simulink model "Assignment2_NaturalPulseDetect"  (R2017b)
settings: Solver=FixedStepAuto  StartTime=0.0  StopTime=inf  FixedStep=0.001  RelTol=1e-3  EnableMultiTasking=on
undefined symbols (not defined in the file): D0, D1, D10, D11, D12, D13, D2, D3, D5, D6, D8, D9, PTA0, PTA1, PTA2, PTB9, PTC16, PTC17, PTC2, PTC4, PTD0, PTD1, PTD2, PTD3
libraries: frdmk64flib x28, etargetslib x7
settings Model: ExtModeTrigDuration=5  Creator=montema2  LastModifiedBy=farona
settings OptimizationCC: PassReuseOutputArgsAs=Individual arguments  MaxStackSize=64
settings DebuggingCC: ParameterTunabilityLossMsg=error
settings HardwareCC: ProdBitPerPointer=32  ProdBitPerSizeT=32  ProdBitPerPtrDiffT=32  ProdLargestAtomicInteger=Long  ProdLargestAtomicFloat=Double  ProdWordSize=32  ProdHWDeviceType=ARM Compatible->ARM Cortex
settings SFSimCC: MATLABDynamicMemAlloc=off
settings RTWCC: SystemTargetFile=ert.tlc  HardwareBoard=NXP FRDM-K64F  TemplateMakefile=ert_default_tmf  GenerateReport=on  Toolchain=GNU Tools for ARM Embedded Processors  IncludeHyperlinkInReport=on  LaunchReport=on  GenerateTraceInfo=on  GenerateTraceReport=on  GenerateTraceReportSl=on  GenerateTraceReportSf=on  GenerateTraceReportEml=on
settings CodeAppCC: ForceParamTrailComments=on  IgnoreCustomStorageClasses=off  OperatorAnnotations=on  SimulinkDataObjDesc=on  SFDataObjDesc=on  InsertBlockDesc=on

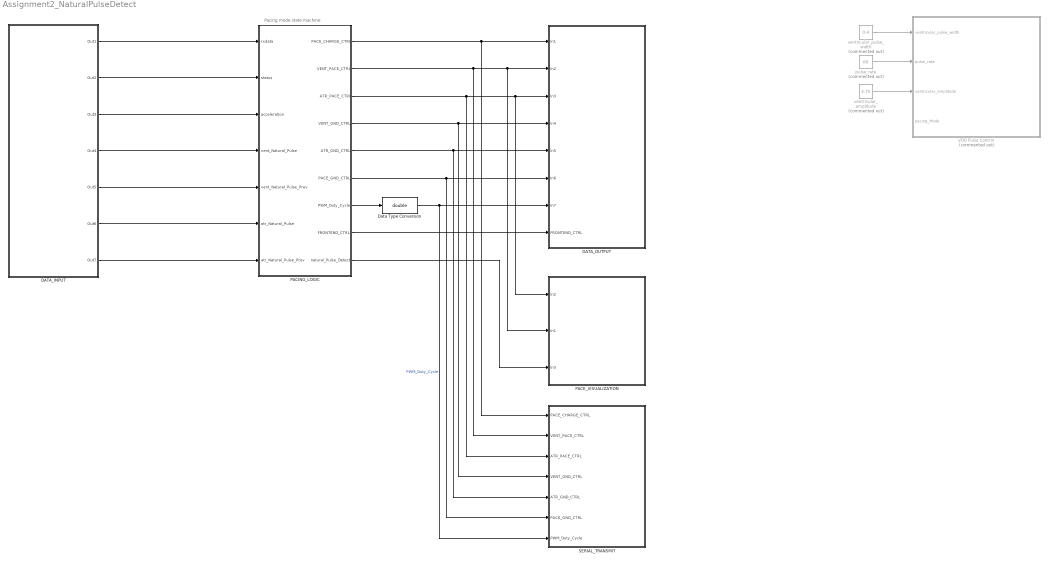
== system Assignment2_NaturalPulseDetect ==
  note: Pacing mode state machine
  DATA_INPUT : Subsystem
  DATA_OUTPUT : Subsystem
  Data Type Conversion : DataTypeConversion  OutDataTypeStr=double  RndMeth=Nearest
  PACE_VISUALIZATION : Subsystem
  PACING_LOGIC : Stateflow chart  TreatAsAtomicUnit=on
  SERIAL_TRANSMIT : Subsystem
  VOO Pulse Control : Subsystem  Commented=on
  pulse_rate : Constant  Commented=on  Value=60  OutMin=[50]  OutMax=[175]
  ventricular_amplitude : Constant  Commented=on  Value=3.75
  ventricular_pulse_width : Constant  Commented=on  Value=0.4
  wires:
  ventricular_pulse_width/1 -> VOO Pulse Control/1(ventricular_pulse_width)
  pulse_rate/1 -> VOO Pulse Control/2(pulse_rate)
  ventricular_amplitude/1 -> VOO Pulse Control/3(ventricular_amplitude)
  PACING_LOGIC/4(VENT_GND_CTRL) -> SERIAL_TRANSMIT/4(VENT_GND_CTRL), DATA_OUTPUT/4(In4)
  PACING_LOGIC/6(PACE_GND_CTRL) -> SERIAL_TRANSMIT/6(PACE_GND_CTRL), DATA_OUTPUT/6(In6)
  PACING_LOGIC/1(PACE_CHARGE_CTRL) -> SERIAL_TRANSMIT/1(PACE_CHARGE_CTRL), DATA_OUTPUT/1(In1)
  PACING_LOGIC/7(PWM_Duty_Cycle) -> Data Type Conversion/1
  PACING_LOGIC/5(ATR_GND_CTRL) -> SERIAL_TRANSMIT/5(ATR_GND_CTRL), DATA_OUTPUT/5(In5)
  PACING_LOGIC/2(VENT_PACE_CTRL) -> SERIAL_TRANSMIT/2(VENT_PACE_CTRL), PACE_VISUALIZATION/2(In1), DATA_OUTPUT/2(In2)
  PACING_LOGIC/3(ATR_PACE_CTRL) -> SERIAL_TRANSMIT/3(ATR_PACE_CTRL), PACE_VISUALIZATION/1(In2), DATA_OUTPUT/3(In3)
  PACING_LOGIC/9(natural_Pulse_Detect) -> PACE_VISUALIZATION/3(In3)
  Data Type Conversion/1 -> SERIAL_TRANSMIT/7(PWM_Duty_Cycle), DATA_OUTPUT/7(In7)  "PWM_Duty_Cycle"
  PACING_LOGIC/8(FRONTEND_CTRL) -> DATA_OUTPUT/8(FRONTEND_CTRL)
  DATA_INPUT/1(Out1) -> PACING_LOGIC/1(rxdata)
  DATA_INPUT/2(Out2) -> PACING_LOGIC/2(status)
  DATA_INPUT/3(Out3) -> PACING_LOGIC/3(acceleration)
  DATA_INPUT/4(Out4) -> PACING_LOGIC/4(vent_Natural_Pulse)
  DATA_INPUT/5(Out5) -> PACING_LOGIC/5(vent_Natural_Pulse_Prev)
  DATA_INPUT/6(Out6) -> PACING_LOGIC/6(atr_Natural_Pulse)
  DATA_INPUT/7(Out7) -> PACING_LOGIC/7(atr_Natural_Pulse_Prev)

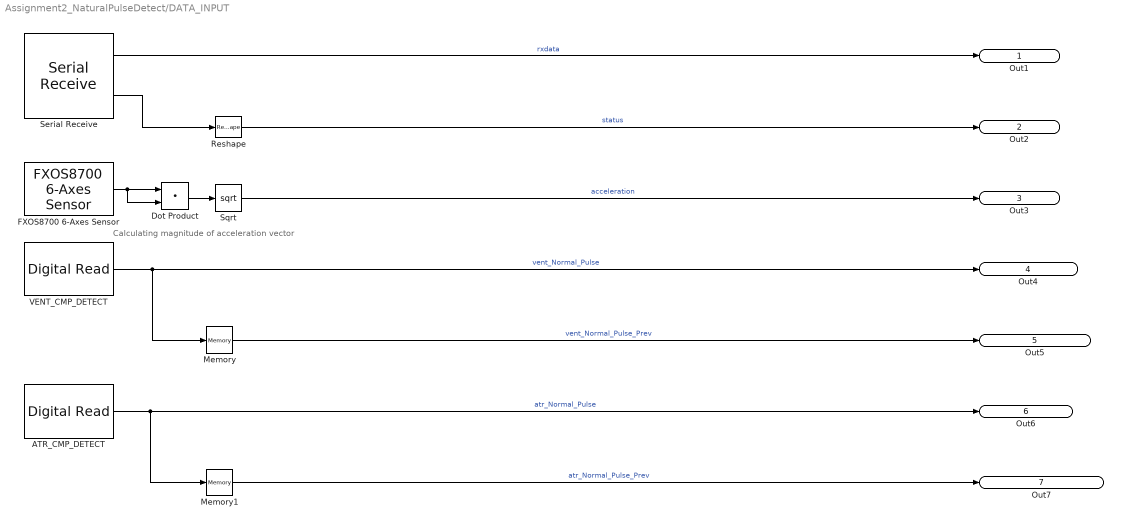
== system Assignment2_NaturalPulseDetect/DATA_INPUT ==
  note: Calculating magnitude of acceleration vector
  ATR_CMP_DETECT : frdmk64flib/Digital Read  Whichpin=PTC16 (D0)  SampleTime=-1
      settings: SourceProductName=Simulink Coder Support Package for NXP FRDM-K64F Board
  Dot Product : DotProduct  InputSameDT=on  OutDataTypeStr=Inherit: Inherit via internal rule
  FXOS8700 6-Axes Sensor : frdmk64flib/FXOS8700 6-Axes Sensor  Activesensor=Accelerometer only  ODR=800Hz  HybridODR=400Hz  Accelfullrange=-2g to +2g  SampleTime=-1
      settings: SourceProductName=Simulink Coder Support Package for NXP FRDM-K64F Board
  Memory : Memory
  Memory1 : Memory
  Reshape : Reshape  OutputDimensionality=Customize  OutputDimensions=[1]
  Serial Receive : frdmk64flib/Serial Receive  SCIModule=0  Baudrate=uint32(9600)  Parity=None  StopBits=1  HardwareFlowControl=None  ByteOrder=LittleEndian  DataType=uint8  DataLength=44  BlockingMode=off  OutputStatus=on  SampleTime=-1
      settings: SourceProductName=Simulink Coder Support Package for NXP FRDM-K64F Board
  Sqrt : Sqrt  SaturateOnIntegerOverflow=on
  VENT_CMP_DETECT : frdmk64flib/Digital Read  Whichpin=PTC17 (D1)  SampleTime=-1
      settings: SourceProductName=Simulink Coder Support Package for NXP FRDM-K64F Board
  Out1 : Outport
  Out2 : Outport  Port=2
  Out3 : Outport  Port=3
  Out4 : Outport  Port=4
  Out5 : Outport  Port=5
  Out6 : Outport  Port=6
  Out7 : Outport  Port=7
  wires:
  Serial Receive/2 -> Reshape/1
  Serial Receive/1 -> Out1/1  "rxdata"
  Dot Product/1 -> Sqrt/1
  FXOS8700 6-Axes Sensor/1 -> Dot Product/2, Dot Product/1
  Reshape/1 -> Out2/1  "status"
  Sqrt/1 -> Out3/1  "acceleration"
  VENT_CMP_DETECT/1 -> Out4/1, Memory/1  "vent_Normal_Pulse"
  Memory/1 -> Out5/1  "vent_Normal_Pulse_Prev"
  Memory1/1 -> Out7/1  "atr_Normal_Pulse_Prev"
  ATR_CMP_DETECT/1 -> Out6/1, Memory1/1  "atr_Normal_Pulse"

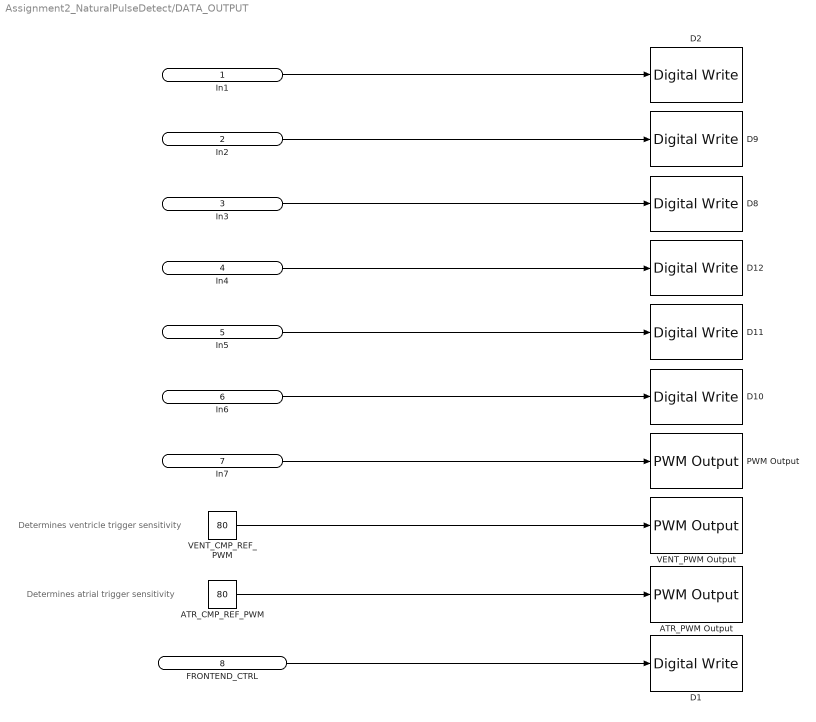
== system Assignment2_NaturalPulseDetect/DATA_OUTPUT ==
  note: Determines ventricle trigger sensitivity
  note: Determines atrial trigger sensitivity
  In1 : Inport
  In2 : Inport  Port=2
  In3 : Inport  Port=3
  In4 : Inport  Port=4
  In5 : Inport  Port=5
  In6 : Inport  Port=6
  In7 : Inport  Port=7
  FRONTEND_CTRL : Inport  Port=8
  ATR_CMP_REF_PWM : Constant  Value=80
  ATR_PWM Output : frdmk64flib/PWM Output  Whichpin=PTC2 (D6)  InitialFrequency=1000  InitialDutyCycle=0
      settings: SourceProductName=Simulink Coder Support Package for NXP FRDM-K64F Board
  D1 : frdmk64flib/Digital Write  Whichpin=PTD1 (D13)
      settings: SourceProductName=Simulink Coder Support Package for NXP FRDM-K64F Board
  D10 : frdmk64flib/Digital Write  Whichpin=PTD0 (D10)
      settings: SourceProductName=Simulink Coder Support Package for NXP FRDM-K64F Board
  D11 : frdmk64flib/Digital Write  Whichpin=PTD2 (D11)
      settings: SourceProductName=Simulink Coder Support Package for NXP FRDM-K64F Board
  D12 : frdmk64flib/Digital Write  Whichpin=PTD3 (D12)
      settings: SourceProductName=Simulink Coder Support Package for NXP FRDM-K64F Board
  D2 : frdmk64flib/Digital Write  Whichpin=PTB9 (D2)
      settings: SourceProductName=Simulink Coder Support Package for NXP FRDM-K64F Board
  D8 : frdmk64flib/Digital Write  Whichpin=PTA0 (D8)
      settings: SourceProductName=Simulink Coder Support Package for NXP FRDM-K64F Board
  D9 : frdmk64flib/Digital Write  Whichpin=PTC4 (D9)
      settings: SourceProductName=Simulink Coder Support Package for NXP FRDM-K64F Board
  PWM Output : frdmk64flib/PWM Output  Whichpin=PTA2 (D5)  InitialFrequency=1000  InitialDutyCycle=0
      settings: SourceProductName=Simulink Coder Support Package for NXP FRDM-K64F Board
  VENT_CMP_REF_PWM : Constant  Value=80
  VENT_PWM Output : frdmk64flib/PWM Output  Whichpin=PTA1 (D3)  InitialFrequency=1000  InitialDutyCycle=0
      settings: SourceProductName=Simulink Coder Support Package for NXP FRDM-K64F Board
  wires:
  In1/1 -> D2/1
  In6/1 -> D10/1
  In2/1 -> D9/1
  In4/1 -> D12/1
  In3/1 -> D8/1
  In7/1 -> PWM Output/1
  In5/1 -> D11/1
  VENT_CMP_REF_PWM/1 -> VENT_PWM Output/1
  FRONTEND_CTRL/1 -> D1/1
  ATR_CMP_REF_PWM/1 -> ATR_PWM Output/1

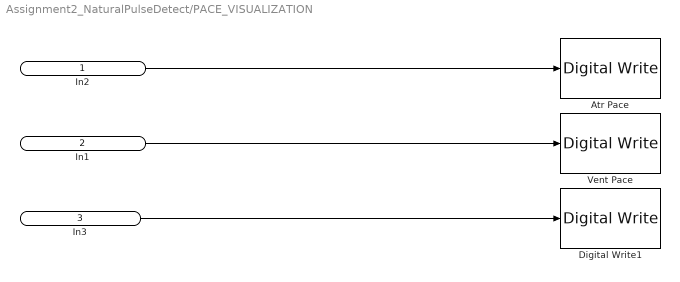
== system Assignment2_NaturalPulseDetect/PACE_VISUALIZATION ==
  In2 : Inport
  In1 : Inport  Port=2
  In3 : Inport  Port=3
  Atr Pace : frdmk64flib/Digital Write  Whichpin=GREEN_LED
      settings: SourceProductName=Simulink Coder Support Package for NXP FRDM-K64F Board
  Digital Write1 : frdmk64flib/Digital Write  Whichpin=BLUE_LED
      settings: SourceProductName=Simulink Coder Support Package for NXP FRDM-K64F Board
  Vent Pace : frdmk64flib/Digital Write  Whichpin=RED_LED
      settings: SourceProductName=Simulink Coder Support Package for NXP FRDM-K64F Board
  wires:
  In3/1 -> Digital Write1/1
  In2/1 -> Atr Pace/1
  In1/1 -> Vent Pace/1

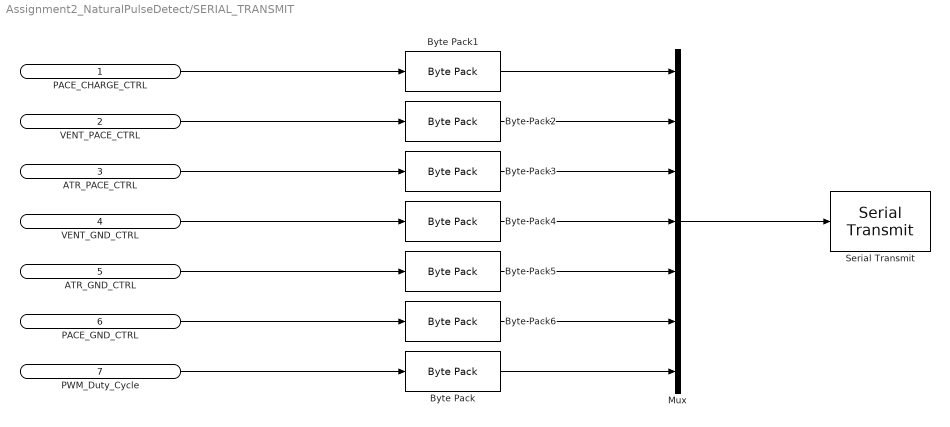
== system Assignment2_NaturalPulseDetect/SERIAL_TRANSMIT ==
  PACE_CHARGE_CTRL : Inport  OutDataTypeStr=boolean
  VENT_PACE_CTRL : Inport  Port=2  OutDataTypeStr=boolean
  ATR_PACE_CTRL : Inport  Port=3  OutDataTypeStr=boolean
  VENT_GND_CTRL : Inport  Port=4  OutDataTypeStr=boolean
  ATR_GND_CTRL : Inport  Port=5  OutDataTypeStr=boolean
  PACE_GND_CTRL : Inport  Port=6  OutDataTypeStr=boolean
  PWM_Duty_Cycle : Inport  Port=7  OutDataTypeStr=double
  Byte Pack : etargetslib/Byte Pack  datatypes={'double'}  byteAlign=1
  Byte Pack{1..6} (6 alike) : etargetslib/Byte Pack  datatypes={'boolean'}  byteAlign=1
  Mux : Mux  Inputs=7
  Serial Transmit : frdmk64flib/Serial Transmit  SCIModule=0  Baudrate=uint32(9600)  Parity=None  StopBits=1  HardwareFlowControl=None  ByteOrder=LittleEndian  BlockingMode=on  OutputStatus=off
      settings: SourceProductName=Simulink Coder Support Package for NXP FRDM-K64F Board
  wires:
  Mux/1 -> Serial Transmit/1
  PACE_CHARGE_CTRL/1 -> Byte Pack1/1
  PWM_Duty_Cycle/1 -> Byte Pack/1
  Byte Pack/1 -> Mux/7
  Byte Pack1/1 -> Mux/1
  VENT_PACE_CTRL/1 -> Byte Pack2/1
  ATR_PACE_CTRL/1 -> Byte Pack3/1
  VENT_GND_CTRL/1 -> Byte Pack4/1
  ATR_GND_CTRL/1 -> Byte Pack5/1
  PACE_GND_CTRL/1 -> Byte Pack6/1
  Byte Pack2/1 -> Mux/2
  Byte Pack3/1 -> Mux/3
  Byte Pack4/1 -> Mux/4
  Byte Pack5/1 -> Mux/5
  Byte Pack6/1 -> Mux/6

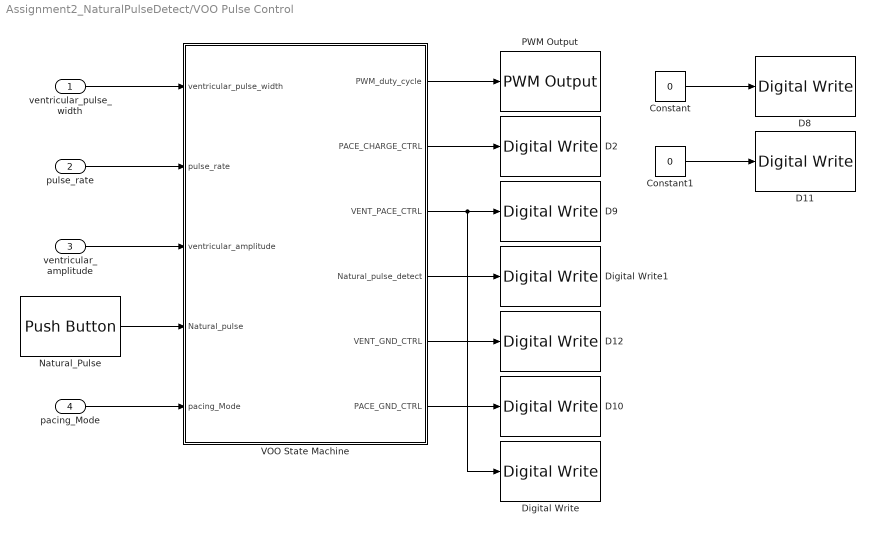
== system Assignment2_NaturalPulseDetect/VOO Pulse Control ==
  ventricular_pulse_width : Inport
  pulse_rate : Inport  Port=2
  ventricular_amplitude : Inport  Port=3
  pacing_Mode : Inport  Port=4
  Constant : Constant  Value=0
  Constant1 : Constant  Value=0
  D10 : frdmk64flib/Digital Write  Whichpin=PTD0 (D10)
      settings: SourceProductName=Simulink Coder Support Package for NXP FRDM-K64F Board
  D11 : frdmk64flib/Digital Write  Whichpin=PTD2 (D11)
      settings: SourceProductName=Simulink Coder Support Package for NXP FRDM-K64F Board
  D12 : frdmk64flib/Digital Write  Whichpin=PTD3 (D12)
      settings: SourceProductName=Simulink Coder Support Package for NXP FRDM-K64F Board
  D2 : frdmk64flib/Digital Write  Whichpin=PTB9 (D2)
      settings: SourceProductName=Simulink Coder Support Package for NXP FRDM-K64F Board
  D8 : frdmk64flib/Digital Write  Whichpin=PTA0 (D8)
      settings: SourceProductName=Simulink Coder Support Package for NXP FRDM-K64F Board
  D9 : frdmk64flib/Digital Write  Whichpin=PTC4 (D9)
      settings: SourceProductName=Simulink Coder Support Package for NXP FRDM-K64F Board
  Digital Write : frdmk64flib/Digital Write  Whichpin=RED_LED
      settings: SourceProductName=Simulink Coder Support Package for NXP FRDM-K64F Board
  Digital Write1 : frdmk64flib/Digital Write  Whichpin=BLUE_LED
      settings: SourceProductName=Simulink Coder Support Package for NXP FRDM-K64F Board
  Natural_Pulse : frdmk64flib/Push Button  Whichswitch=SW2  SampleTime1=-1
      settings: SourceProductName=Simulink Coder Support Package for NXP FRDM-K64F Board
  PWM Output : frdmk64flib/PWM Output  Whichpin=PTA2 (D5)  InitialFrequency=1000  InitialDutyCycle=0
      settings: SourceProductName=Simulink Coder Support Package for NXP FRDM-K64F Board
  VOO State Machine : Stateflow chart  TreatAsAtomicUnit=on
  wires:
  ventricular_pulse_width/1 -> VOO State Machine/1(ventricular_pulse_width)
  VOO State Machine/1(PWM_duty_cycle) -> PWM Output/1
  VOO State Machine/3(VENT_PACE_CTRL) -> Digital Write/1, D9/1
  pulse_rate/1 -> VOO State Machine/2(pulse_rate)
  VOO State Machine/2(PACE_CHARGE_CTRL) -> D2/1
  VOO State Machine/5(VENT_GND_CTRL) -> D12/1
  VOO State Machine/6(PACE_GND_CTRL) -> D10/1
  Constant/1 -> D8/1
  Constant1/1 -> D11/1
  Natural_Pulse/1 -> VOO State Machine/4(Natural_pulse)
  VOO State Machine/4(Natural_pulse_detect) -> Digital Write1/1
  ventricular_amplitude/1 -> VOO State Machine/3(ventricular_amplitude)
  pacing_Mode/1 -> VOO State Machine/5(pacing_Mode)

== stateflow chart Assignment2_NaturalPulseDetect/PACING_LOGIC ==
  state INITIAL
    %Set intial values of parameters
    %VOO mode?
    entry: rateAdapt = 0;
    vent_Pulse_Width = 10; %milliseconds
    atr_Pulse_Width = 10;
    min_Rate_Lim = 60; %bpm
    vent_Pulse_Amp = 3.5; %volts
    atr_Pulse_Amp = 3.5;
  state VENT_PACEING
    state VENT_CURRENT_IN
      entry:PWM_Duty_Cycle = vent_Pulse_Amp;
      PACE_CHARGE_CTRL=false;
      VENT_GND_CTRL=false;
      VENT_PACE_CTRL=true;
    state VENT_CURRENT_OUT
      entry:
      VENT_PACE_CTRL=false;
      PACE_CHARGE_CTRL=true;
      VENT_GND_CTRL=true;
    VENT_CURRENT_OUT -> VENT_CURRENT_IN [order 3] : [(pace_Mode == 1 || pace_Mode ==3 || pace_Mode == 7 || pace_Mode == 9)&&(after((60000/min_Rate_Lim)-(vent_Pulse_Width),msec))]
    VENT_CURRENT_IN -> VENT_CURRENT_OUT : [after((vent_Pulse_Width),msec)]
  state STANDBY
    %Wait for signal from DCM
  state VENTRICLE_INIT
    entry:VENT_PACE_CTRL=false;
    VENT_GND_CTRL=true;
    ATR_PACE_CTRL=false;
    ATR_GND_CTRL=true;
    PACE_CHARGE_CTRL=true;
    PACE_GND_CTRL=true;
  note: Serial recieve standby loop
  note: double check ATR_GND_CTRL state
  state VENT_NATURAL_PACE_SENSING
    state NP_VENT_CHARGE
      entry:
      VENT_PACE_CTRL=false;
      PACE_CHARGE_CTRL=true;
      VENT_GND_CTRL=true;
    state VENT_PULSE_SENSE
      entry: natural_Pulse_Detect = true;
      exit: natural_Pulse_Detect = false;
    NP_VENT_CHARGE -> VENT_PULSE_SENSE [order 1] : [vent_Natural_Pulse==true && vent_Natural_Pulse_Prev==false && after(PVARP,msec)]
    VENT_PULSE_SENSE -> NP_VENT_CHARGE
  note: Check if pace mode is valid
  note: double check VENT_GND_CTRL state
  state PARAM_INIT1
    entry: pace_Mode = typecast(rxdata(1:2), 'int16');
    min_Rate_Lim = typecast(rxdata(3:4), 'int16');
    max_Rate_Lim = typecast(rxdata(5:6), 'int16');
    max_Sensor_Rate = typecast(rxdata(7:8), 'int16');
    fix_AV_Delay = typecast(rxdata(9:10), 'int16');
    vent_Pulse_Amp = (typecast(rxdata(11:14), 'single')/5)*100;
    atr_Pulse_Amp = (typecast(rxdata(15:18), 'single')/5)*100;
    vent_Pulse_Width = typecast(rxdata(19:20), 'int16');
    atr_Pulse_Width = typecast(rxdata(21:22), 'int16');
    vent_Sens = typecast(rxdata(23:26), 'single');
    atr_Sens = typecast(rxdata(27:30), 'single');
    vent_Ref_Per = typecast(rxdata(31:32), 'int16');
    atr_Ref_Per = typecast(rxdata(33:34), 'int16');
    PVARP = typecast(rxdata(35:36), 'int16');
    activity_Thresh = typecast(rxdata(37:38), 'int16');
    reaction_Time = typecast(rxdata(39:40), 'int16');
    response_Factor = typecast(rxdata(41:42), 'int16');
    recovery_Time = typecast(rxdata(43:44), 'int16');
  note: Determine if mode is rate adaptive
  state PARAM_INIT [commented out]
    entry: pace_Mode = typecast(rxdata(1:2), 'int16');
    min_Rate_Lim = typecast(rxdata(3:4), 'int16');
    max_Rate_Lim = typecast(rxdata(5:6), 'int16');
    max_Sensor_Rate = typecast(rxdata(7:8), 'int16');
    fix_AV_Delay = typecast(rxdata(9:10), 'int16');
    vent_Pulse_Amp = (typecast(rxdata(11:14), 'single')/5)*100;
    atr_Pulse_Amp = (typecast(rxdata(15:18), 'single')/5)*100;
    vent_Pulse_Width = typecast(rxdata(19:20), 'int16');
    atr_Pulse_Width = typecast(rxdata(21:22), 'int16');
    vent_Sens = typecast(rxdata(23:26), 'single');
    atr_Sens = typecast(rxdata(27:30), 'single');
    vent_Ref_Per = typecast(rxdata(31:32), 'int16');
    atr_Ref_Per = typecast(rxdata(33:34), 'int16');
    PVARP = typecast(rxdata(35:36), 'int16');
    activity_Thresh = typecast(rxdata(37:38), 'int16');
    reaction_Time = typecast(rxdata(39:40), 'int16');
    response_Factor = typecast(rxdata(41:42), 'int16');
    recovery_Time = typecast(rxdata(43:44), 'int16');
    %current_Rate = typecast(min_Rate_Lim, 'double');
    current_Accel = acceleration;
  state SENS_CTRL
    state SENS_TRUE
      entry: FRONTEND_CTRL = 1;
    state SENS_FALSE
      entry: FRONTEND_CTRL = 0;
    SENS_TRUE -> (junction 191)
    (junction 187) -> SENS_TRUE [order 1] : [pace_Mode == 3 || pace_Mode == 4 || pace_Mode == 6 || pace_Mode == 9 || pace_Mode == 10 || pace_Mode == 12]
    (junction 187) -> SENS_FALSE [order 2]
    SENS_FALSE -> (junction 191)
  state ATR_PACEING
    state ATR_CURRENT_IN
      entry:PWM_Duty_Cycle = atr_Pulse_Amp;
      PACE_CHARGE_CTRL=false;
      ATR_GND_CTRL=false;
      ATR_PACE_CTRL=true;
    state ATR_CURRENT_OUT
      entry:
      ATR_PACE_CTRL=false;
      PACE_CHARGE_CTRL=true;
      ATR_GND_CTRL=true;
    ATR_CURRENT_OUT -> ATR_CURRENT_IN [order 2] : [(pace_Mode == 2 || pace_Mode == 4 || pace_Mode == 8 || pace_Mode == 10)&&(after((60000/min_Rate_Lim)-(atr_Pulse_Width),msec))]
    ATR_CURRENT_IN -> ATR_CURRENT_OUT : [after((atr_Pulse_Width),msec)]
  state ATRIAL_INIT
    entry:VENT_PACE_CTRL=false;
    VENT_GND_CTRL=true;
    ATR_PACE_CTRL=false;
    ATR_GND_CTRL=true;
    PACE_CHARGE_CTRL=true;
    PACE_GND_CTRL=true;
  state ATR_NATURAL_PACE_SENSING
    state NP_ATR_CHARGE
      entry:
      ATR_PACE_CTRL=false;
      PACE_CHARGE_CTRL=true;
      ATR_GND_CTRL=true;
    state ATR_PULSE_SENSE
      entry: natural_Pulse_Detect = true;
      exit: natural_Pulse_Detect = false;
    NP_ATR_CHARGE -> ATR_PULSE_SENSE [order 1] : [atr_Natural_Pulse==true && atr_Natural_Pulse_Prev==false && after(PVARP,msec)]
    ATR_PULSE_SENSE -> NP_ATR_CHARGE
  state Rate_Adaptive_Mode [commented out]
    state Rate_Adapt_INIT [commented out]
      entry:
      react_Time_Intrvl = (max_Sensor_Rate - min_Rate_Lim)/(typecast(reaction_Time, 'double'));
      rec_Time_Intrvl = (max_Sensor_Rate - min_Rate_Lim)/(typecast(recovery_Time, 'double'));
    note: Yes
    note: Yes
    state Rate_Is_Max [commented out]
      entry:
      curent_rate = max_Sensor_Rate;
    note: Yes
    state Increase_Current_Rate [commented out]
      entry:
      current_Rate = current_Rate + react_Time_Intrvl;
    Rate_Adapt_INIT -> (junction 138) [commented out] : [current_Accel > activity_Thresh]
    (junction 138) -> (junction 140) [commented out] : [(current_Rate + response_Factor) > max_Sensor_Rate]
    (junction 140) -> Rate_Is_Max [commented out]
    (junction 140) -> Increase_Current_Rate [commented out] : [(current_Rate + react_Time_Intrvl) < max_Sensor_Rate]
    Rate_Is_Max -> ? [commented out] : [x == 3]
  state DUAL_INIT
    entry:VENT_PACE_CTRL=false;
    VENT_GND_CTRL=true;
    ATR_PACE_CTRL=false;
    ATR_GND_CTRL=true;
    PACE_CHARGE_CTRL=true;
    PACE_GND_CTRL=true;
  state DDD_INIT
    %For assignment 3
  VENTRICLE_INIT -> VENT_PULSE_SENSE [order 1] : [FRONTEND == 1 && vent_Natural_Pulse==true && vent_Natural_Pulse_Prev==false]
  NP_VENT_CHARGE -> VENT_CURRENT_IN [order 2] : [(pace_Mode == 1 || pace_Mode ==3 || pace_Mode == 7 || pace_Mode == 9)&&(after((60000/min_Rate_Lim)-(vent_Pulse_Width),msec))]
  ATR_CURRENT_OUT -> ATR_PULSE_SENSE [order 4] : [FRONTEND == 1 && atr_Natural_Pulse==true && atr_Natural_Pulse_Prev==false && after(atr_Pulse_Width, msec)]
  NP_ATR_CHARGE -> ATR_CURRENT_IN [order 2] : [(pace_Mode == 2 || pace_Mode == 4 || pace_Mode == 8 || pace_Mode == 10)&&(after((60000/min_Rate_Lim)-(atr_Pulse_Width),msec))]
  NP_VENT_CHARGE -> ATR_CURRENT_IN [order 3] : [(pace_Mode ==  5 || pace_Mode ==11)&&(after((60000/min_Rate_Lim)-(vent_Pulse_Width)-(atr_Pulse_Width)-(fix_AV_Delay),msec))]
  NP_ATR_CHARGE -> VENT_CURRENT_IN [order 3] : [(pace_Mode ==  5 || pace_Mode ==11)&&(after((fix_AV_Delay),msec))]
  VENT_CURRENT_OUT -> VENT_PULSE_SENSE [order 2] : [FRONTEND == 1 && vent_Natural_Pulse==true && vent_Natural_Pulse_Prev==false && after(vent_Pulse_Width, msec)]
  (junction 191) -> (junction 7)
  (default) -> INITIAL
  INITIAL -> STANDBY
  (junction 7) -> STANDBY [order 5]
  VENTRICLE_INIT -> VENT_CURRENT_IN [order 2] : [after((60000/min_Rate_Lim),msec)]
  ATR_CURRENT_OUT -> VENT_CURRENT_IN [order 3] : [(pace_Mode ==  5 || pace_Mode ==11)&&(after((fix_AV_Delay),msec))]
  (junction 5) -> STANDBY [order 2]
  STANDBY -> (junction 5) : [status == 0]
  (junction 7) -> VENTRICLE_INIT [order 1] : [pace_Mode ==1 || pace_Mode == 3 || pace_Mode ==7 || pace_Mode == 9]
  (junction 179) -> (junction 5)
  (junction 5) -> (junction 38) [order 1] : [typecast(rxdata(1:2), 'int16') >= 0 && typecast(rxdata(1:2), 'int16') <= 12]
  (junction 38) -> PARAM_INIT1
  ATRIAL_INIT -> ATR_CURRENT_IN [order 2] : [after((60000/min_Rate_Lim),msec)]
  ATRIAL_INIT -> ATR_PULSE_SENSE [order 1] : [FRONTEND == 1 && atr_Natural_Pulse==true && atr_Natural_Pulse_Prev==false]
  (junction 176) -> (junction 179)
  VENT_CURRENT_OUT -> (junction 176) [order 1] : [status == 0]
  ATR_CURRENT_OUT -> (junction 176) [order 1] : [status == 0]
  PARAM_INIT1 -> (junction 183) [order 1] : [pace_Mode <=5]{rateAdapt = 0}
  (junction 183) -> (junction 187)
  PARAM_INIT1 -> (junction 183) [order 2] : [pace_Mode > 6]{rateAdapt = 1}
  (junction 7) -> ATRIAL_INIT [order 2] : [pace_Mode ==2 || pace_Mode == 4 || pace_Mode ==8 || pace_Mode ==10]
  (junction 7) -> DDD_INIT [order 4] : [pace_Mode ==6 || pace_Mode ==12 ]
  (junction 7) -> DUAL_INIT [order 3] : [pace_Mode ==5 || pace_Mode == 11]
  VENT_CURRENT_OUT -> ATR_CURRENT_IN [order 4] : [(pace_Mode ==  5 || pace_Mode ==11)&&(after((60000/min_Rate_Lim)-(vent_Pulse_Width)-(atr_Pulse_Width)-(fix_AV_Delay),msec))]
  DUAL_INIT -> ATR_CURRENT_IN : [after((60000/min_Rate_Lim),msec)]
  DDD_INIT -> ATR_CURRENT_IN : [after((60000/min_Rate_Lim),msec)]
  data: rxdata input uint8; status input uint8; PACE_CHARGE_CTRL output boolean; VENT_PACE_CTRL output boolean; ATR_PACE_CTRL output boolean; VENT_GND_CTRL output boolean; ATR_GND_CTRL output boolean; PACE_GND_CTRL output boolean; PWM_Duty_Cycle output single; natural_Pace local; atr_Sens local single; PVARP local int16; activity_Thresh local int16; recovery_Time local int16; response_Factor local int16; reaction_Time local int16; max_Rate_Lim local int16; max_Sensor_Rate local int16; vent_Ref_Per local int16; vent_Sens local single; atr_Ref_Per local int16; rateAdapt local; pace_Mode local int16; fix_AV_Delay local int16; atr_Pulse_Width local int16; vent_Pulse_Width local int16; min_Rate_Lim local int16; vent_Pulse_Amp local single; atr_Pulse_Amp local single; current_Rate local double; current_Accel local double; acceleration input double; react_Time_Intrvl local double; rec_Time_Intrvl local double; FRONTEND_CTRL output int8; vent_Natural_Pulse input boolean; vent_Natural_Pulse_Prev input boolean; natural_Pulse_Detect output; atr_Natural_Pulse input boolean; atr_Natural_Pulse_Prev input boolean

== stateflow chart Assignment2_NaturalPulseDetect/VOO Pulse Control/VOO State Machine ==
  note: Switch States:
      | true=closed
      | false=open
  state current_into_heart
    entry:
    PACE_CHARGE_CTRL=false;
    VENT_GND_CTRL=false;
    VENT_PACE_CTRL=true;
  state start_state
    entry:VENT_PACE_CTRL=false;
    VENT_GND_CTRL=true;
    PACE_CHARGE_CTRL=true;
    PACE_GND_CTRL=true;
    PWM_duty_cycle=((ventricular_amplitude/5)*100);
  state current_out_of_heart
    entry:
    VENT_PACE_CTRL=false;
    PACE_CHARGE_CTRL=true;
    VENT_GND_CTRL=true;
  state natural_pace
    entry: Natural_pulse_detect=true;
    exit: Natural_pulse_detect=false;
  (default) -> start_state
  start_state -> current_into_heart [order 1] : [after(((60/pulse_rate)*1000),msec)]
  current_into_heart -> natural_pace [order 2] : [Natural_pulse==true]
  start_state -> natural_pace [order 2] : [Natural_pulse==true]
  natural_pace -> start_state : [Natural_pulse==false]
  current_into_heart -> current_out_of_heart [order 1] : [after((ventricular_pulse_width),msec)]
  current_out_of_heart -> current_into_heart [order 1] : [after(((60/pulse_rate)*1000)-(ventricular_pulse_width),msec)]
  current_out_of_heart -> natural_pace [order 2] : [Natural_pulse==true]
  data: ventricular_pulse_width input double; pulse_rate input double; ventricular_amplitude input double; PWM_duty_cycle output double [0..100]; PACE_CHARGE_CTRL output boolean; VENT_PACE_CTRL output boolean; Natural_pulse_detect output; VENT_GND_CTRL output boolean; PACE_GND_CTRL output boolean; Natural_pulse input boolean; pacing_Mode input uint8
